simulink model "closedLoop"  (R2021b)
settings: Solver=VariableStepAuto  StartTime=0.0  StopTime=500  RelTol=1e-3
undefined symbols (not defined in the file or in its folder): sigbuilder_block
libraries: slpidlib x1
settings Model: Creator=Asus  LastModifiedBy=Asus

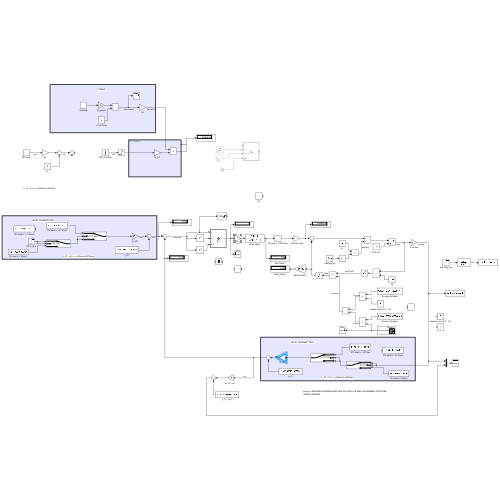
[thumbnail: Simulink's stored preview of the top-level diagram]
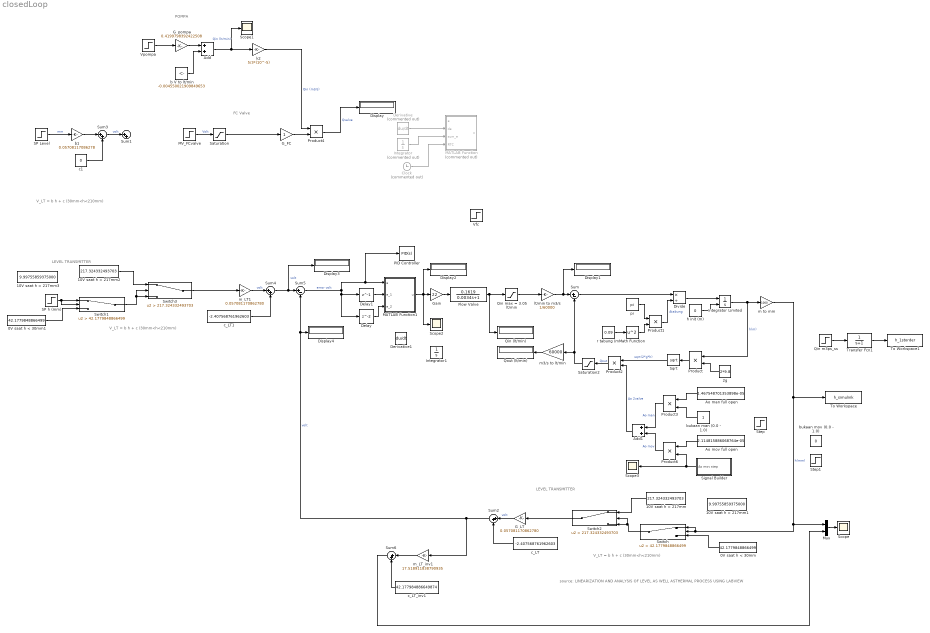
== system closedLoop ==
  note: V_LT = b h + c (30mm<h<210mm)
  note: LEVEL TRANSMITTER
  note: FC Valve
  note: POMPA
  note: source: LINEARIZATION AND ANALYSIS OF LEVEL AS WELL ASTHERMAL PROCESS USING LABVIEW
  note: V_LT = b h + c (30mm<h<210mm)
  note: LEVEL TRANSMITTER
  note: V_LT = b h + c (30mm<h<210mm)
  0V saat h < 30mm : Constant  Value=42.1779848866499
  0V saat h < 30mm1 : Constant  Value=42.1779848866499
  10V saat h > 217mm : Constant  Value=217.324332493703
  10V saat h > 217mm1 : Constant  Value=9.99755859375000
  10V saat h > 217mm2 : Constant  Value=217.324332493703
  10V saat h > 217mm3 : Constant  Value=9.99755859375000
  2g : Constant  Value=2*9.8
  Add : Sum
  Add1 : Sum
  Ao man full open : Constant  Value=1.467548701353898e-05
  Ao mov full open : Constant  Value=2.114815886068764e-05
  Clock : Clock  Commented=on
  Delay : Delay  InitialCondition=0
  Delay1 : Delay  DelayLength=1  InitialCondition=0
  Derivative : Derivative  Commented=on
  Derivative1 : Derivative
  Display{,1..4} (5 alike) : Display
  Divide : Product  Inputs=*/
  Flow Valve : TransferFcn  Numerator=[0.1619]  Denominator=[0.0034 1]
  G_FC : Gain
  G_LT : Gain  Gain=0.057081170862780
  G_pompa : Gain  Gain=0.4199798392422508
  Gain : Gain  Gain=22
  Integrator : Integrator  Commented=on
  Integrator Limited : Integrator  InitialConditionSource=external  LimitOutput=on  UpperSaturationLimit=1  LowerSaturationLimit=0
  Integrator1 : Integrator
  MATLAB Function : MATLAB Function  Commented=on  TreatAsAtomicUnit=on
  MATLAB Function1 : MATLAB Function  TreatAsAtomicUnit=on
  MV_FCvalve : Step  SampleTime=0
  Math Function : Math  Operator=square  SaturateOnIntegerOverflow=on
  Mux : Mux  Inputs=2
  PID Controller : slpidlib/PID Controller  Controller=PID  Form=Parallel  TimeDomain=Continuous-time  UseExternalTs=off  SampleTime=-1  IntegratorMethod=Forward Euler  FilterMethod=Forward Euler  ControllerParametersSource=internal  P=10  I=0.1  D=0  UseFilter=on  N=100  TunerSelectOption=Transfer Function Based (PID Tuner App)  InitialConditionSource=internal  InitialConditionForIntegrator=0  InitialConditionForFilter=0  DifferentiatorICPrevScaledInput=0  ExternalReset=none  TrackingMode=off  Kt=1  LimitOutput=on  SatLimitsSource=internal  UpperSaturationLimit=22  LowerSaturationLimit=0  LinearizeAsGain=on  AntiWindupMode=none  Kb=1  POutMin=[]  POutMax=[]  IOutMin=[]  IOutMax=[]  DOutMin=[]  DOutMax=[]  NOutMin=[]  NOutMax=[]  SumOutMin=[]  SumOutMax=[]  SaturationOutMin=[]  SaturationOutMax=[]  PParamMin=[]  PParamMax=[]  IParamMin=[]  IParamMax=[]  DParamMin=[]  DParamMax=[]  NParamMin=[]  NParamMax=[]  KbParamMin=[]  KbParamMax=[]  KtParamMin=[]  KtParamMax=[]  KbOutMin=[]  KbOutMax=[]  KtOutMin=[]  KtOutMax=[]  IntegratorOutMin=[]  IntegratorOutMax=[]  FilterOutMin=[]  FilterOutMax=[]  SumI1OutMin=[]  SumI1OutMax=[]  SumI2OutMin=[]  SumI2OutMax=[]  SumI3OutMin=[]  SumI3OutMax=[]  SumI4OutMin=[]  SumI4OutMax=[]  SumDOutMin=[]  SumDOutMax=[]  DifferentiatorOutMin=[]  DifferentiatorOutMax=[]  FilterDiffOutCoefMin=[]  FilterDiffOutCoefMax=[]  ReciprocalOutMin=[]  ReciprocalOutMax=[]  SumDenOutMin=[]  SumDenOutMax=[]  SumNumOutMin=[]  SumNumOutMax=[]  DivideOutMin=[]  DivideOutMax=[]  UdiffTsProdOutMin=[]  UdiffTsProdOutMax=[]  NTsProdOutMin=[]  NTsProdOutMax=[]  UintegralTsProdOutMin=[]  UintegralTsProdOutMax=[]  UngainTsProdOutMin=[]  UngainTsProdOutMax=[]  IntegratorContinuousStateAttributes=''  IntegratorStateMustResolveToSignalObject=off  IntegratorRTWStateStorageClass=Auto  FilterContinuousStateAttributes=''  FilterStateMustResolveToSignalObject=off  FilterRTWStateStorageClass=Auto  ParallelPVariant=InternalParameters  IdealPVariant=Disabled  IVariant=InternalParameters  DVariant=InternalParameters  IntegratorVariant=Continuous  SatVariant=Enabled  AWVariant=Passthrough  PCopyVariant=Disabled  TRVariant=Disabled  FdbkBlocksVariant=Forward  IdealPFdbkVariant=Disabled  SatFdbkVariant=Disabled  DerivativeFilterVariant=ContFilter  NVariant=InternalParameters  NCopyVariant=Disabled  FilterICVariant=InternalICsFilter  IntegratorICVariant=InternalICs  ExternalResetVariant=Disabled  TRSumVariant=Passthrough  SumFdbkVariant=Disabled  SumVariant=Sum_PID  TsampFilterVariant=InternalTs  TsampNgainVariant=Passthrough  TsampIntegralVariant=Passthrough  ExternalSaturationOutDataTypeStr=Inherit: Same as second input
  Product{,1..4,6} (6 alike) : Product
  Qin (lt/min) : Display
  Qin m3ps_ss : Step  After=1.613207956317757e-05  SampleTime=0
  Qin max = 3.05 lt/min : Saturate  UpperLimit=3.05  LowerLimit=0
  Qout (lt/min) : Display
  SP Level : Step  SampleTime=0
  SP h (mm) : Step  Time=0  After=200  SampleTime=0.05
  Saturation : Saturate  UpperLimit=10  LowerLimit=0
  Saturation2 : Saturate
  Scope{,1..3} (4 alike) : Scope
  Signal Builder : Subsystem  Tag=STV Subsys  LoadFcn=sigbuilder_block('load');  StartFcn=sigbuilder_block('start');  StopFcn=sigbuilder_block('stop');  ClipboardFcn=sigbuilder_block('clipboard');  mask(Sigbuilder block){tuvar=[0:10]}
      mask help: Simulink:masks:SigbuilderBlock_MD
      mask init:
      | if ~strcmp(get_param(bdroot(gcbh),'SimulationStatus'),'stopped') tuvar = sigbuilder_block('maskInit'); end
      settings: CopyFcn=sigbuilder_block('copy');  DeleteFcn=sigbuilder_block('delete');  ModelCloseFcn=sigbuilder_block('modelClose');  PreSaveFcn=sigbuilder_block('preSave');  PauseFcn=sigbuilder_block('pause');  ContinueFcn=sigbuilder_block('continue');  NameChangeFcn=sigbuilder_block('namechange');  OpenFcn=sigbuilder_block('open',[292.8 50.4 550.8 400.2 ]);  CloseFcn=sigbuilder_block('close');
      mask Display: plot(0, 0, 100, 100,[2, 2, 32, 32, 2], [68, 8, 8, 68, 68],[32, 2], [38, 38], [32, 19, 2],[53, 60, 44], [32, 17, 17, 2],[16, 16, 31, 31]);txt = getActiveGroup(gcbh);text(2, 100, txt,'verticalAlignment', 'top');
  Sqrt : Sqrt  SaturateOnIntegerOverflow=on
  Step : Step  Time=300  SampleTime=0
  Step1 : Step  Time=300  SampleTime=0
  Sum : Sum  Inputs=|+-
  Sum{1..4,6} (5 alike) : Sum  Inputs=|++
  Sum5 : Sum  Inputs=|+-
  Switch : Switch  Criteria=u2 > Threshold  Threshold=42.1779848866499
  Switch1 : Switch  Criteria=u2 > Threshold  Threshold=42.1779848866499
  Switch2 : Switch  Criteria=u2 > Threshold  Threshold=217.324332493703
  Switch3 : Switch  Criteria=u2 > Threshold  Threshold=217.324332493703
  To Workspace : ToWorkspace  VariableName=h_simulink  SampleTime=-1
      settings: Save2DSignal=2-D array (concatenate along first dimension)
  To Workspace1 : ToWorkspace  VariableName=h_1storder  SampleTime=-1
      settings: Save2DSignal=2-D array (concatenate along first dimension)
  Transfer Fcn1 : TransferFcn  Denominator=[1 1]
  Vfc : Step  After=5.9792  SampleTime=0
  Vpompa : Step  After=10  SampleTime=0
  b V to lt/min : Constant  Value=-0.004550021909849653
  b1 : Gain  Gain=0.05708117086278
  bukaan man (0.0 - 1.0) : Constant
  bukaan mov (0.0 - 1.0) : Constant  Value=0
  c1 : Constant  Value=0
  c_LT : Constant  Value=-2.407568761962603
  c_LT1 : Constant  Value=-2.407568761962603
  c_LT_inv1 : Constant  Value=42.177984886649874
  h init (m) : Constant  Value=0
  k2 : Gain  Gain=5/3*(10^-5)
  lt/min to m3/s : Gain  Gain=1/60000
  m to mm : Gain  Gain=1000
  m3/s to lt/min : Gain  Gain=60000
  m_LT1 : Gain  Gain=0.057081170862780
  m_LT_inv1 : Gain  Gain=17.518911838790935
  pi : Constant  Value=pi
  r tabung (m) : Constant  Value=0.09
  wires:
  Divide/1 -> Integrator Limited/1
  Product/1 -> Sqrt/1
  2g/1 -> Product/2
  Sqrt/1 -> Product2/1  "sqrt(2*g*h)"
  h init (m)/1 -> Integrator Limited/2
  Product1/1 -> Divide/2  "Atabung"
  pi/1 -> Product1/1
  Math Function/1 -> Product1/2
  r tabung (m)/1 -> Math Function/1
  Add1/1 -> Product2/2  "Ao 2valve"
  G_pompa/1 -> Add/1
  Add/1 -> Scope1/1, k2/1  "Qin (lt/min)"
  b V to lt/min/1 -> Add/2
  k2/1 -> Product4/1  "Qin (m3/s)"
  Product4/1 -> Display/1  "Qvalve"
  MV_FCvalve/1 -> Saturation/1  "Volt"
  G_FC/1 -> Product4/2
  SP Level/1 -> b1/1  "mm"
  b1/1 -> Sum3/1
  Integrator Limited/1 -> Product/1, m to mm/1  "h(m)"
  m to mm/1 -> To Workspace/1, Mux/1, Switch/1, Switch/2  "h(mm)"
  Vpompa/1 -> G_pompa/1
  Saturation/1 -> G_FC/1
  0V saat h < 30mm/1 -> Switch/3
  Switch/1 -> Switch2/2, Switch2/3
  10V saat h > 217mm/1 -> Switch2/1
  Switch2/1 -> G_LT/1
  G_LT/1 -> Sum2/1  "volt"
  c_LT/1 -> Sum2/2
  c1/1 -> Sum3/2
  Sum3/1 -> Sum1/1  "volt"
  Mux/1 -> Scope/1
  Ao man full open/1 -> Product3/1
  Product3/1 -> Add1/1  "Ao man"
  Product6/1 -> Add1/2  "Ao mov"
  Ao mov full open/1 -> Product6/1
  Sum/1 -> Divide/1
  Product2/1 -> Saturation2/1  "Qout"
  Clock/1 -> MATLAB Function/4(RTC)
  Integrator/1 -> MATLAB Function/3(sum_e)
  Derivative/1 -> MATLAB Function/2(de)
  Flow Valve/1 -> Qin max = 3.05 lt/min/1, Qin (lt/min)/1
  lt/min to m3/s/1 -> Display1/1, Sum/1
  Sum5/1 -> Delay/1, Delay1/1, PID Controller/1, MATLAB Function1/1(e)  "error volt"
  Qin m3ps_ss/1 -> Transfer Fcn1/1
  Transfer Fcn1/1 -> To Workspace1/1
  m_LT_inv1/1 -> Sum6/1
  Sum2/1 -> m_LT_inv1/1, Sum5/2, Display4/1  "volt"
  c_LT_inv1/1 -> Sum6/2
  Switch3/1 -> m_LT1/1
  Switch1/1 -> Switch3/2, Switch3/3
  m_LT1/1 -> Sum4/1  "volt"
  c_LT1/1 -> Sum4/2
  0V saat h < 30mm1/1 -> Switch1/3
  10V saat h > 217mm2/1 -> Switch3/1
  Sum4/1 -> Display3/1, Sum5/1  "volt"
  SP h (mm)/1 -> Switch1/1, Switch1/2
  Sum6/1 -> Mux/2
  Delay1/1 -> MATLAB Function1/2(e_1)
  Delay/1 -> MATLAB Function1/3(e_2)
  bukaan man (0.0 - 1.0)/1 -> Product3/2
  Gain/1 -> Flow Valve/1
  MATLAB Function1/1(u) -> Scope2/1, Display2/1, Gain/1
  Signal Builder/1(Ao mov step) -> Scope3/1, Product6/2
  m3/s to lt/min/1 -> Qout (lt/min)/1
  Qin max = 3.05 lt/min/1 -> lt/min to m3/s/1
  Saturation2/1 -> Sum/2, m3/s to lt/min/1

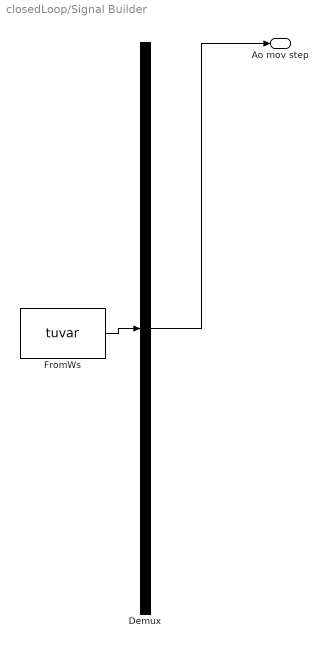
== system closedLoop/Signal Builder ==
  Demux : Demux  Tag=STV Demux  Outputs=1
      settings: DisplayOption=none
  FromWs : FromWorkspace  Tag=STV FromWs  VariableName=tuvar
      SigBuilderData=|
      | common.afterFinalStr = 'Extrapolate'
      | common.sampleTime = 0
      | dataSet.timeRange = [0 1000]
      | dataSet.name = 'Group 1'
      | sbobj.Groups.Name = 'Group 1'
      | sbobj.Groups.Signals.Name = 'Ao mov step'
      | sbobj.Groups.Signals.XData = [0 200 200 400 400 600 600 800 800 1000]
      | sbobj.Groups.Signals.YData = [0 0 0.5 0.5 1 1 0.5 0.5 0 0]
      | sbobj.Groups.TimeRange = [0 1000]
  Ao mov step : Outport  Tag=STV Outport
  wires:
  Demux/1 -> Ao mov step/1
  FromWs/1 -> Demux/1

== matlab function closedLoop/MATLAB Function1 ==
  settings: updateMethod=DISCRETE
  data: u output; e input; e_1 input; e_2 input
function u = fcn(e, e_1, e_2)
    % initial condition
    persistent w_input v_hidden y_hidden delta2 hj ei_1 ei_2  lr n
    if isempty(w_input)
%         w_input = zeros(3,3);
        w_input = rand(3,3);
        n = 0;
    end
    if isempty(v_hidden)
%         v_hidden = zeros(1,3);
        v_hidden = rand(1,3);
    end
    if isempty(delta2)
        delta2 = zeros(1,3);
    end
    if isempty(hj)
        hj = [0;0;0];
    end
    if isempty(ei_1)
        ei_1 = 0;
    end
    if isempty(ei_2)
        ei_2 = 0;
    end
    if isempty(lr)
        lr = 0.01;
    end
    ei = e
    x_input = [e; e_1; e_2];
    % FORWARD PROPAGATION
    % Input layer to hidden layer
    for j_hiddenLayer = 1:3
        Sj = w_input(j_hiddenLayer,:) * x_input; % summing hidden neuron ke-j
        hj(j_hiddenLayer) = 1/(1 + exp(-1*Sj));
    end
    % hidden layer to output layer
    r = v_hidden * hj;
    u = 1/(1+exp(-1*r));

    % BACKWARD PROPAGATION: RETROPROPAGATION
    alpha = 0.008;
    lr = lr + alpha*abs(ei);
%     lr = 0.001;
%     MSE = 0.5*(e_1^2)
    delta1 = ei*u*(1-u);
%     dey_deu = sign(ei);
    dey_deu = 1; %sign(ei);
    for j_hiddenLayer = 1:3
        v_hidden(j_hiddenLayer) = v_hidden(j_hiddenLayer) + lr * dey_deu * delta1 * hj(j_hiddenLayer);
        delta2(j_hiddenLayer) = delta1 * v_hidden(j_hiddenLayer) * hj(j_hiddenLayer) * (1 - hj(j_hiddenLayer));
        
        for i_inputLayer = 1:3
            w_input(j_hiddenLayer,i_inputLayer) = w_input(j_hiddenLayer,i_inputLayer) + lr * dey_deu * delta2(j_hiddenLayer) * x_input(i_inputLayer);
        end
    end
    
    ei_2 = ei_1;
    ei_1 = ei;
    w_input
    v_hidden
    n = n + 1

== matlab function closedLoop/MATLAB Function ==
  data: e input; u output; de input; sum_e input; RTC input
function u = fcn(e, de, sum_e, RTC)
RTC
u = 100*e + 200*sum_e + 1*de;
